simulink model "modele_detaille_algorithme_LIMA_MILITAO_PINHEIRO"  (R2019a)
settings: Solver=ode45  StartTime=0.0  StopTime=8  RelTol=1e-4  EnableMultiTasking=on
undefined symbols (not defined in the file): fa, fm, G1, G_den_RST, G_num_RST, Ja, Jm, Jt, ka, kt, R, R1, ro, S, T, Te, tsim
settings Model: Creator=xshi  LastModifiedBy=dougl
settings DataIOCC: LimitDataPoints=on  SaveFormat=Array  SignalLoggingSaveFormat=ModelDataLogs  ReturnWorkspaceOutputs=off  SignalLoggingName=sigsOut
settings DebuggingCC: SaveWithParameterizedLinksMsg=none  UnderspecifiedInitializationDetection=Classic  MergeDetectMultiDrivingBlocksExec=none  SignalResolutionControl=TryResolveAllWithWarning  MultiTaskDSMMsg=warning  MultiTaskCondExecSysMsg=none
settings HardwareCC: ProdBitPerPointer=32  ProdBitPerSizeT=32  ProdBitPerPtrDiffT=32  ProdLargestAtomicFloat=None  ProdIntDivRoundTo=Undefined  ProdEndianess=Unspecified  ProdWordSize=32  ProdHWDeviceType=32-bit Generic  TargetBitPerPointer=64  TargetBitPerSizeT=64  TargetBitPerPtrDiffT=64  TargetLongLongMode=on  TargetIntDivRoundTo=Zero  TargetEndianess=LittleEndian  TargetWordSize=64  TargetHWDeviceType=MATLAB Host  ProdEqTarget=off
settings ModelReferenceCC: PropagateSignalLabelsOutOfModel=off
settings GRTTargetCC: CombineOutputUpdateFcns=off  GRTInterface=on
settings ConfigComp: CovMetricSettings=dw  CovSaveCumulativeToWorkspaceVar=on  CovSaveSingleToWorkspaceVar=on

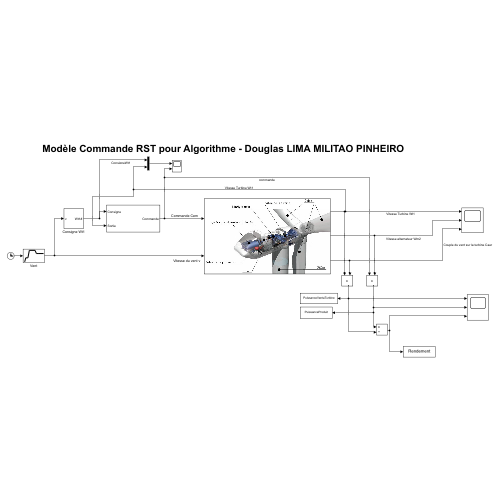
[thumbnail: Simulink's stored preview of the top-level diagram]
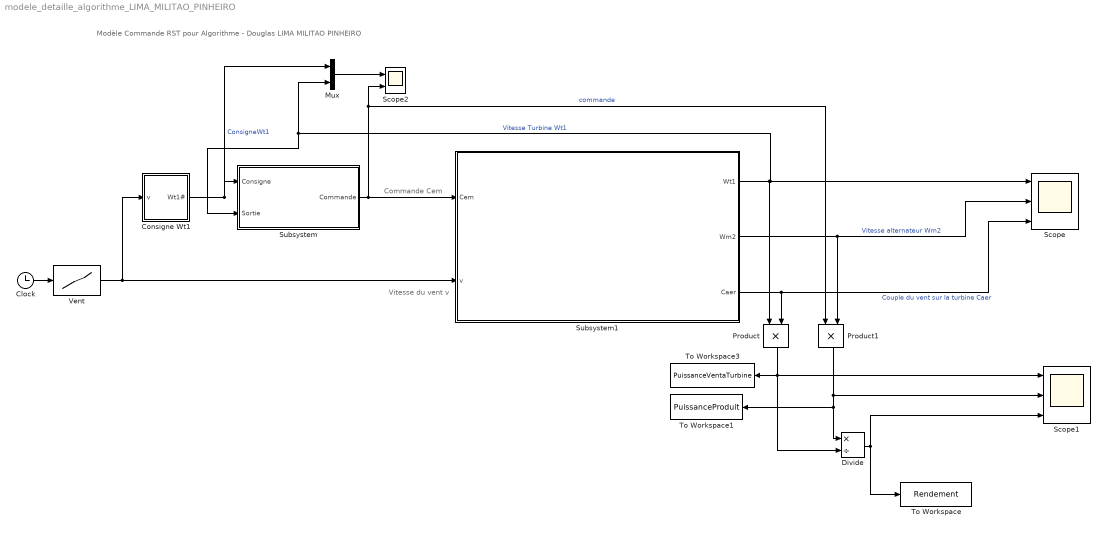
== system modele_detaille_algorithme_LIMA_MILITAO_PINHEIRO ==
  note: Vitesse du vent v
  note: Commande Cem
  note: Modèle Commande RST pour Algorithme - Douglas LIMA MILITAO PINHEIRO
  Clock : Clock
  Consigne Wt1 : Subsystem
  Divide : Product  Inputs=*/
  Mux : Mux  Inputs=2
  Product : Product
  Product1 : Product
  Scope : Scope  NumInputPorts=3
  Scope1 : Scope  NumInputPorts=3
  Scope2 : Scope  NumInputPorts=2
  Subsystem : Subsystem
  Subsystem1 : Subsystem
      mask Display:
      | image('eolienne.jpg');
      | %port_label('output', 1, 'référence vitesse turbine');
      | %port_label('output', 2, 'vitesse turbine');
      | %port_label('output', 3, 'vitesse alternateur');
      | %port_label('input', 1, 'Vitese du vent v');
      | %port_label('input', 2, 'Commande Cem');
  To Workspace : ToWorkspace  VariableName=Rendement  SampleTime=tsim
  To Workspace1 : ToWorkspace  VariableName=PuissanceProduit  SampleTime=tsim
  To Workspace3 : ToWorkspace  VariableName=PuissanceVentaTurbine  SampleTime=tsim
  Vent : Lookup  InputValues="[0 0.1 0.6 1.5 2 4.5 5  6  8]"  Table=[0 0 5 5 14 14 10 10 10]  SaturateOnIntegerOverflow=on
  wires:
  Clock/1 -> Vent/1
  Vent/1 -> Subsystem1/2(v), Consigne Wt1/1(v)
  Consigne Wt1/1(Wt1#) -> Mux/1, Subsystem/1(Consigne)  "ConsigneWt1"
  Subsystem1/2(Wm2) -> Product1/2, Scope/2  "Vitesse alternateur Wm2"
  Subsystem1/3(Caer) -> Product/2, Scope/3  "Couple du vent sur la turbine Caer"
  Subsystem1/1(Wt1) -> Scope/1, Mux/2, Subsystem/2(Sortie), Product/1  "Vitesse Turbine Wt1"
  Mux/1 -> Scope2/1
  Subsystem/1(Commande) -> Subsystem1/1(Cem), Product1/1, Scope2/2  "commande"
  Product/1 -> Divide/2, To Workspace3/1, Scope1/1
  Product1/1 -> To Workspace1/1, Divide/1, Scope1/2
  Divide/1 -> Scope1/3, To Workspace/1

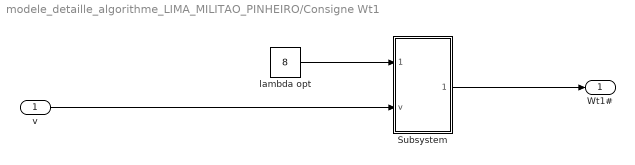
== system modele_detaille_algorithme_LIMA_MILITAO_PINHEIRO/Consigne Wt1 ==
  v : Inport
  Subsystem : Subsystem
  lambda opt : Constant  Value=8
  Wt1# : Outport
  wires:
  lambda opt/1 -> Subsystem/1(Lambda opt)
  v/1 -> Subsystem/2(v)
  Subsystem/1(Wt1#) -> Wt1#/1

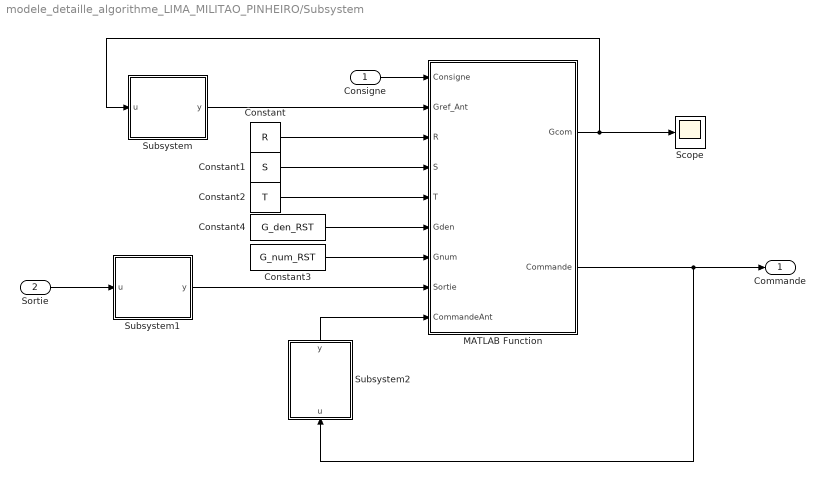
== system modele_detaille_algorithme_LIMA_MILITAO_PINHEIRO/Subsystem ==
  Consigne : Inport
  Sortie : Inport  Port=2
  Constant : Constant  Value=R
  Constant1 : Constant  Value=S
  Constant2 : Constant  Value=T
  Constant3 : Constant  Value=G_num_RST
  Constant4 : Constant  Value=G_den_RST
  MATLAB Function : MATLAB Function  TreatAsAtomicUnit=on
  Scope : Scope
  Subsystem : Subsystem
  Subsystem1 : Subsystem
  Subsystem2 : Subsystem
  Commande : Outport
  wires:
  MATLAB Function/2(Commande) -> Subsystem2/1(u), Commande/1
  Sortie/1 -> Subsystem1/1(u)
  Subsystem/1(y) -> MATLAB Function/2(Gref_Ant)
  Subsystem1/1(y) -> MATLAB Function/8(Sortie)
  Subsystem2/1(y) -> MATLAB Function/9(CommandeAnt)
  Constant/1 -> MATLAB Function/3(R)
  Constant2/1 -> MATLAB Function/5(T)
  Constant1/1 -> MATLAB Function/4(S)
  Constant3/1 -> MATLAB Function/7(Gnum)
  Constant4/1 -> MATLAB Function/6(Gden)
  Consigne/1 -> MATLAB Function/1(Consigne)
  MATLAB Function/1(Gcom) -> Scope/1, Subsystem/1(u)

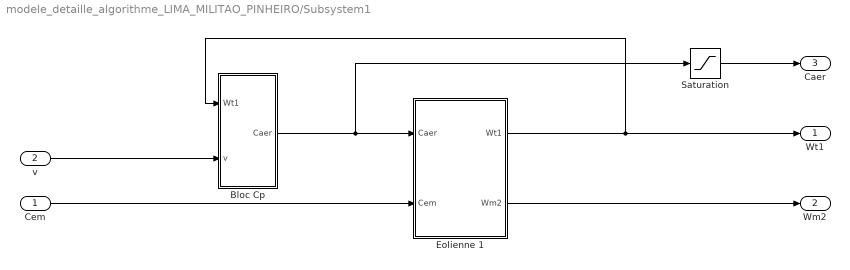
== system modele_detaille_algorithme_LIMA_MILITAO_PINHEIRO/Subsystem1 ==
  Cem : Inport
  v : Inport  Port=2
  Bloc Cp : Subsystem
  Eolienne 1 : Subsystem
  Saturation : Saturate  UpperLimit=50e3  LowerLimit=-50e3
  Wt1 : Outport
  Wm2 : Outport  Port=2
  Caer : Outport  Port=3
  wires:
  Eolienne 1/1(Wt1) -> Wt1/1, Bloc Cp/1(Wt1)
  v/1 -> Bloc Cp/2(v)
  Bloc Cp/1(Caer) -> Saturation/1, Eolienne 1/1(Caer)
  Cem/1 -> Eolienne 1/2(Cem)
  Eolienne 1/2(Wm2) -> Wm2/1
  Saturation/1 -> Caer/1

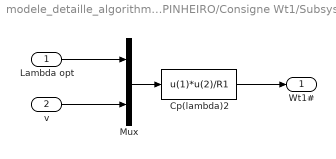
== system modele_detaille_algorithme_LIMA_MILITAO_PINHEIRO/Consigne Wt1/Subsystem ==
  Lambda opt : Inport
  v : Inport  Port=2
  Cp(lambda)2 : Fcn  Expr=u(1)*u(2)/R1
  Mux : Mux  Inputs=2
  Wt1# : Outport
  wires:
  Mux/1 -> Cp(lambda)2/1
  v/1 -> Mux/2
  Cp(lambda)2/1 -> Wt1#/1
  Lambda opt/1 -> Mux/1

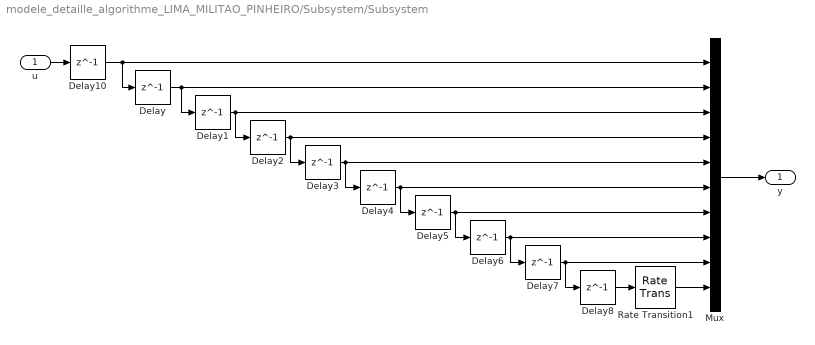
== system modele_detaille_algorithme_LIMA_MILITAO_PINHEIRO/Subsystem/Subsystem ==
  u : Inport
  Delay{,1..8,10} (10 alike) : Delay  DelayLength=1  SampleTime=Te
  Mux : Mux  Inputs=10
  Rate Transition1 : RateTransition  OutPortSampleTime=Te
  y : Outport
  wires:
  Mux/1 -> y/1
  u/1 -> Delay10/1
  Delay/1 -> Mux/2, Delay1/1
  Delay1/1 -> Mux/3, Delay2/1
  Delay2/1 -> Mux/4, Delay3/1
  Delay3/1 -> Mux/5, Delay4/1
  Delay4/1 -> Mux/6, Delay5/1
  Delay5/1 -> Mux/7, Delay6/1
  Delay6/1 -> Mux/8, Delay7/1
  Delay7/1 -> Delay8/1, Mux/9
  Delay8/1 -> Rate Transition1/1
  Delay10/1 -> Mux/1, Delay/1
  Rate Transition1/1 -> Mux/10

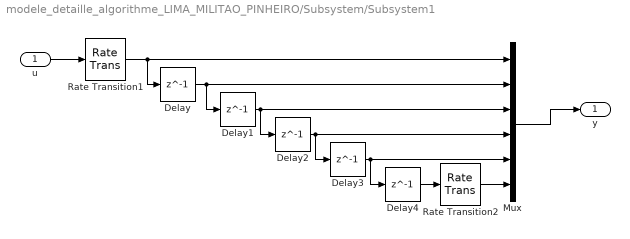
== system modele_detaille_algorithme_LIMA_MILITAO_PINHEIRO/Subsystem/Subsystem1 ==
  u : Inport
  Delay{,1..4} (5 alike) : Delay  DelayLength=1  SampleTime=Te
  Mux : Mux  Inputs=6
  Rate Transition1 : RateTransition  OutPortSampleTime=Te
  Rate Transition2 : RateTransition  OutPortSampleTime=Te
  y : Outport
  wires:
  Delay2/1 -> Delay3/1, Mux/4
  Delay1/1 -> Delay2/1, Mux/3
  Delay/1 -> Delay1/1, Mux/2
  Rate Transition1/1 -> Delay/1, Mux/1
  Mux/1 -> y/1
  Delay3/1 -> Delay4/1, Mux/5
  u/1 -> Rate Transition1/1
  Delay4/1 -> Rate Transition2/1
  Rate Transition2/1 -> Mux/6

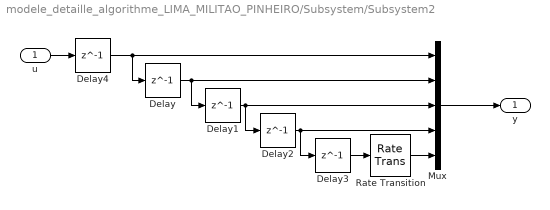
== system modele_detaille_algorithme_LIMA_MILITAO_PINHEIRO/Subsystem/Subsystem2 ==
  u : Inport
  Delay{,1..4} (5 alike) : Delay  DelayLength=1  SampleTime=Te
  Mux : Mux  Inputs=5
  Rate Transition : RateTransition  OutPortSampleTime=Te
  y : Outport
  wires:
  Mux/1 -> y/1
  u/1 -> Delay4/1
  Delay/1 -> Mux/2, Delay1/1
  Delay1/1 -> Mux/3, Delay2/1
  Delay2/1 -> Mux/4, Delay3/1
  Delay3/1 -> Rate Transition/1
  Delay4/1 -> Mux/1, Delay/1
  Rate Transition/1 -> Mux/5

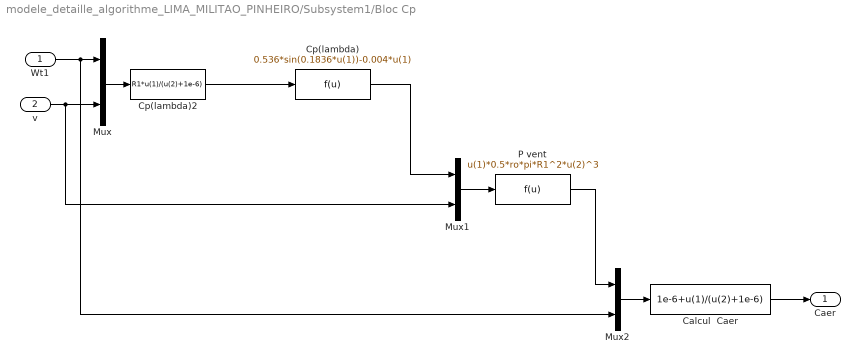
== system modele_detaille_algorithme_LIMA_MILITAO_PINHEIRO/Subsystem1/Bloc Cp ==
  Wt1 : Inport
  v : Inport  Port=2
  Calcul  Caer : Fcn  Expr=1e-6+u(1)/(u(2)+1e-6)
  Cp(lambda) : Fcn  Expr=0.536*sin(0.1836*u(1))-0.004*u(1)
  Cp(lambda)2 : Fcn  Expr=R1*u(1)/(u(2)+1e-6)
  Mux : Mux  Inputs=2
  Mux1 : Mux  Inputs=2
  Mux2 : Mux  Inputs=2
  P vent : Fcn  Expr=u(1)*0.5*ro*pi*R1^2*u(2)^3
  Caer : Outport
  wires:
  Mux/1 -> Cp(lambda)2/1
  Cp(lambda)2/1 -> Cp(lambda)/1
  Wt1/1 -> Mux/1, Mux2/2
  Cp(lambda)/1 -> Mux1/1
  v/1 -> Mux/2, Mux1/2
  Mux1/1 -> P vent/1
  P vent/1 -> Mux2/1
  Mux2/1 -> Calcul  Caer/1
  Calcul  Caer/1 -> Caer/1

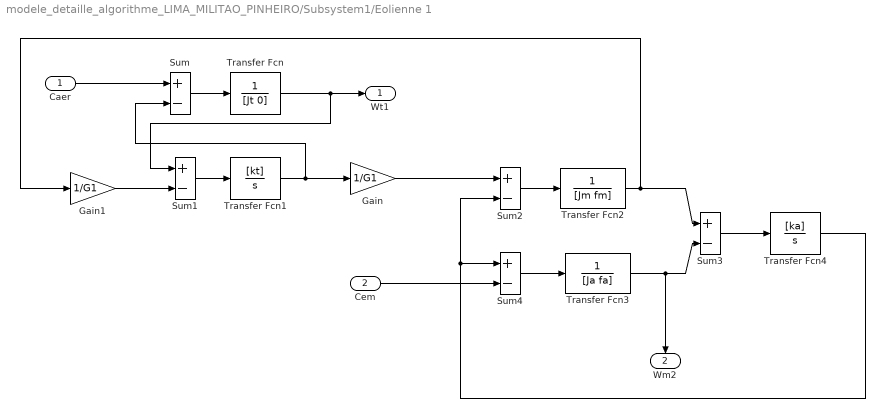
== system modele_detaille_algorithme_LIMA_MILITAO_PINHEIRO/Subsystem1/Eolienne 1 ==
  Caer : Inport
  Cem : Inport  Port=2
  Gain : Gain  Gain=1/G1  SaturateOnIntegerOverflow=on  OutDataTypeStr=Inherit: Same as input  ParamDataTypeStr=Inherit: Same as input
  Gain1 : Gain  Gain=1/G1  SaturateOnIntegerOverflow=on  OutDataTypeStr=Inherit: Same as input  ParamDataTypeStr=Inherit: Same as input
  Sum{,1..4} (5 alike) : Sum  Inputs=+-  SaturateOnIntegerOverflow=on
  Transfer Fcn : TransferFcn  Denominator=[Jt 0]
  Transfer Fcn1 : TransferFcn  Numerator=[kt]  Denominator=[1 0]
  Transfer Fcn2 : TransferFcn  Denominator=[Jm fm]
  Transfer Fcn3 : TransferFcn  Denominator=[Ja fa]
  Transfer Fcn4 : TransferFcn  Numerator=[ka]  Denominator=[1 0]
  Wt1 : Outport
  Wm2 : Outport  Port=2
  wires:
  Sum/1 -> Transfer Fcn/1
  Sum1/1 -> Transfer Fcn1/1
  Transfer Fcn1/1 -> Sum/2, Gain/1
  Transfer Fcn/1 -> Sum1/1, Wt1/1
  Gain1/1 -> Sum1/2
  Gain/1 -> Sum2/1
  Sum2/1 -> Transfer Fcn2/1
  Transfer Fcn2/1 -> Sum3/1, Gain1/1
  Transfer Fcn3/1 -> Sum3/2, Wm2/1
  Sum4/1 -> Transfer Fcn3/1
  Sum3/1 -> Transfer Fcn4/1
  Transfer Fcn4/1 -> Sum2/2, Sum4/1
  Cem/1 -> Sum4/2
  Caer/1 -> Sum/1

== matlab function modele_detaille_algorithme_LIMA_MILITAO_PINHEIRO/Subsystem/MATLAB Function ==
  data: Gcom output; Consigne input; Gref_Ant input; Commande output; R input; S input; T input; Gden input; Gnum input; Sortie input; CommandeAnt input
function [Gcom, Commande] = fcn(Consigne, Gref_Ant, R, S, T, Gden, Gnum, Sortie, CommandeAnt)

Gcom = Gden(1)*Consigne - Gnum(2)*Gref_Ant(1);

Tcom = T(1)*Gcom;
Rcom = 0;

for i=2:length(T)
    Tcom = Tcom + T(i)*Gref_Ant(i-1);
end

for i=1:length(R)
    Rcom = Rcom + R(i)*Sortie(i);
end

Commande = Tcom - Rcom;

for i=1:length(CommandeAnt)
    Commande = Commande - S(i+1)*CommandeAnt(i);
end
